simulink model "MPC"  (R2024b)
settings: Solver=ode4  StartTime=0.0  StopTime=tsim  FixedStep=baseRate  RelTol=1e-6  AbsTol=1e-6
values from neighbouring files (symbols this model uses):
  IBLACK = 0.1996    [unpackData.m]
  IRED = 0.1982    [unpackData.m]
  m = m + 5    (= 4)    [unpackData.m]
  M = diag([1/m; 1/m; 1/I])    [unpackData.m]
  mBLACK = 11.3620    (= 11.362)    [unpackData.m]
  mRED = 11.2970    (= 11.297)    [unpackData.m]
  N = 0    [unpackData.m]
  Q = blkdiag(0.0001*eye(2), 0.00001)    [unpackData.m]
  R = diag([6;6;6])    [unpackData.m]
undefined symbols (not defined in the file or in its folder): a1, a2, a3, alpha, alpha_m, alpha_t, alphas, alphas_t, alphat, Am, b, b0, b1, b2, b3, baseRate, Bm, C, c, c1, c1t, c2, c2t, camera_FOV, camera_offset, Cm, d, dataRate, DiscIntNeverNeededParam, Dm, docking_face, docking_offset, drop_states_ARM, drop_states_BLACK, drop_states_BLUE, drop_states_RED, epsilon, epsilont, eta, F_black_X_nominal, F_black_Y_nominal, F_blue_X_nominal, F_blue_Y_nominal, F_max, F_red_X_nominal, F_red_Y_nominal, f_t, F_t, F_thrusters_BLACK, F_thrusters_BLUE, F_thrusters_RED, F_u, f_u, F_v, gamma, Gamma1_el, Gamma1_sh, Gamma1_wr, Gamma2_el, Gamma2_sh ... (+118)
libraries: simulink x33, nvidiaSharedBlocks x13, slpidlib x6, MainLibrary x5, dspsigops x3, dspinverses x3, nvidiaIMUSensorslib x1
(part 5 of 11)

== system MPC/Thruster Control Code/Change BLUE Behavior ==
  note: Calculate the percentage of time each thruster must be on, and send to the PWM blocks.
  note: Using the attitude, rotate the forces into the body frame.
  note: Calculate which thrusters must be turned on and for how long.
  Action Port : ActionPort  ActionPortLabel=if(u1 == 3 | u2 == 1)
  Calculate Duty Cycle : Subsystem
  Data Store Read : DataStoreRead  DataStoreName=BLUE_Controls  IndexOptions=Index vector (dialog)  Indices=1  OutputSizes=1
  Data Store Read1 : DataStoreRead  DataStoreName=BLUE_Measured_States_RAW  IndexOptions=Index vector (dialog)  Indices=1  OutputSizes=1
  Data Store Write3 : DataStoreWrite  DataStoreName=BLUE_Saturated_Controls  IndexOptions=Index vector (dialog)  Indices=1  OutputSizes=1
  Demux : Demux  Outputs=[2,1]
  Demux1 : Demux  Outputs=[2,1,6]
  Mux1 : Mux  Inputs=2
  Rotate Forces to Body : Subsystem
  Terminator : Terminator
  Terminator1 : Terminator
  BLUE DC : Outport  VectorParamsAs1DForOutWhenUnconnected=off
  wires:
  Calculate Duty Cycle/1(Duty Cycle) -> BLUE DC/1
  Rotate Forces to Body/1(F_b) -> Mux1/1
  Demux/2 -> Mux1/2
  Mux1/1 -> Calculate Duty Cycle/1("[Fx_b; Fy_b; Tz]")
  Calculate Duty Cycle/2(Saturated Forces Moments) -> Data Store Write3/1
  Data Store Read/1 -> Demux/1
  Demux/1 -> Rotate Forces to Body/1("F_I ")
  Data Store Read1/1 -> Demux1/1
  Demux1/2 -> Calculate Duty Cycle/2(Measured Attitude), Rotate Forces to Body/2(Rz)
  Demux1/1 -> Terminator/1
  Demux1/3 -> Terminator1/1

== system MPC/Thruster Control Code/Change RED Behavior ==
  note: Calculate which thrusters must be turned on and for how long.
  note: Calculate the percentage of time each thruster must be on, and send to the PWM blocks.
  note: Using the attitude, rotate the forces into the body frame.
  Action Port : ActionPort  ActionPortLabel=if(u1 == 1 | u2 == 1)
  Calculate Duty Cycle : Subsystem
  Data Store Read : DataStoreRead  DataStoreName=RED_Controls  IndexOptions=Index vector (dialog)  Indices=1  OutputSizes=1
  Data Store Read2 : DataStoreRead  DataStoreName=RED_Measured_States_RAW  IndexOptions=Index vector (dialog)  Indices=1  OutputSizes=1
  Data Store Write1 : DataStoreWrite  DataStoreName=RED_Saturated_Controls  IndexOptions=Index vector (dialog)  Indices=1  OutputSizes=1
  Demux : Demux  Outputs=[2,1]
  Demux1 : Demux  Outputs=[2,1,6]
  Mux1 : Mux  Inputs=2
  Rotate Forces to Body : Subsystem
  Terminator : Terminator
  Terminator1 : Terminator
  RED DC : Outport  VectorParamsAs1DForOutWhenUnconnected=off
  wires:
  Demux/1 -> Rotate Forces to Body/1("F_I ")
  Mux1/1 -> Calculate Duty Cycle/1("[Fx_b; Fy_b; Tz]")
  Demux/2 -> Mux1/2
  Demux1/2 -> Calculate Duty Cycle/2(Measured Attitude), Rotate Forces to Body/2(Rz)
  Rotate Forces to Body/1(F_b) -> Mux1/1
  Data Store Read/1 -> Demux/1
  Demux1/1 -> Terminator/1
  Demux1/3 -> Terminator1/1
  Data Store Read2/1 -> Demux1/1
  Calculate Duty Cycle/2(Saturated Forces Moments) -> Data Store Write1/1
  Calculate Duty Cycle/1(Duty Cycle) -> RED DC/1

== system MPC/1 - Experiment Logic/Phase #2: Initial Position/Desired Joint Angles RED ==
  Constant1 : Constant  Value=pi/2
  Constant2 : Constant  Value=0
  Constant3 : Constant  Value=pi/2
  Mux : Mux  Inputs=3
  Target Array : Outport
  wires:
  Mux/1 -> Target Array/1
  Constant3/1 -> Mux/1
  Constant1/1 -> Mux/2
  Constant2/1 -> Mux/3

== system MPC/1 - Experiment Logic/Phase #2: Initial Position/Desired Position BLACK ==
  Desired States (BLACK) : Constant  Value=init_states_BLACK  SampleTime=-1
  Target Array : Outport
  wires:
  Desired States (BLACK)/1 -> Target Array/1

== system MPC/1 - Experiment Logic/Phase #2: Initial Position/Desired Position BLUE ==
  Desired States (BLUE) : Constant  Value=init_states_BLUE  SampleTime=-1
  Target Array : Outport
  wires:
  Desired States (BLUE)/1 -> Target Array/1

== system MPC/1 - Experiment Logic/Phase #2: Initial Position/Desired Position RED ==
  Constant2 : Constant  Value=init_states_RED
  Target Array : Outport
  wires:
  Constant2/1 -> Target Array/1

== system MPC/1 - Experiment Logic/Phase #3: Experiment/Sub-Phase #1 ==
  note: Experiment Logic (BLUE)
  note: Experiment Logic (Robotic Manipulator)
  note: Experiment Logic (RED)
  note: Experiment Logic (BLACK)
  note: Control Blocks
  Action Port : ActionPort  ActionPortLabel=if(u1 < u2)
  Constant : Constant  Value=[0 0 0]
  Constant1 : Constant  Value=[0 0 0]
  Constant{11..12,14..15,18} (5 alike) : Constant  Value=0
  Constant4 : Constant  Value=2
  Constant5 : Constant  Value=3
  Constant6 : Constant
  Constant8 : Constant  Value=2
  Data Store Write1 : DataStoreWrite  DataStoreName=ARM_Path_Planner_Selection  IndexOptions=Index vector (dialog)  Indices=1  OutputSizes=1
  Data Store Write10 : DataStoreWrite  DataStoreName=Toggle_Nav  IndexOptions=Index vector (dialog)  Indices=1  OutputSizes=1
  Data Store Write13 : DataStoreWrite  DataStoreName=ARM_Desired_States  IndexOptions=Index vector (dialog)  Indices=1  OutputSizes=1
  Data Store Write16 : DataStoreWrite  DataStoreName=BLUE_Control_Law_Enabler  IndexOptions=Index vector (dialog)  Indices=1  OutputSizes=1
  Data Store Write18 : DataStoreWrite  DataStoreName=BLUE_Desired_States  IndexOptions=Index vector (dialog)  Indices=1  OutputSizes=1
  Data Store Write2 : DataStoreWrite  DataStoreName=ARM_Control_Law_Enabler  IndexOptions=Index vector (dialog)  Indices=1  OutputSizes=1
  Data Store Write22 : DataStoreWrite  DataStoreName=BLUE_Path_Planner_Selection  IndexOptions=Index vector (dialog)  Indices=1  OutputSizes=1
  Data Store Write23 : DataStoreWrite  DataStoreName=BLACK_Path_Planner_Selection  IndexOptions=Index vector (dialog)  Indices=1  OutputSizes=1
  Data Store Write24 : DataStoreWrite  DataStoreName=RED_Path_Planner_Selection  IndexOptions=Index vector (dialog)  Indices=1  OutputSizes=1
  Data Store Write3 : DataStoreWrite  DataStoreName=RED_Control_Law_Enabler  IndexOptions=Index vector (dialog)  Indices=1  OutputSizes=1
  Data Store Write4 : DataStoreWrite  DataStoreName=BLACK_Control_Law_Enabler  IndexOptions=Index vector (dialog)  Indices=1  OutputSizes=1
  Data Store Write5 : DataStoreWrite  DataStoreName=BLACK_Desired_States  IndexOptions=Index vector (dialog)  Indices=1  OutputSizes=1
  Data Store Write7 : DataStoreWrite  DataStoreName=Float_State  IndexOptions=Index vector (dialog)  Indices=1  OutputSizes=1
  Data Store Write9 : DataStoreWrite  DataStoreName=RED_Desired_States  IndexOptions=Index vector (dialog)  Indices=1  OutputSizes=1
  Desired Position BLACK : Subsystem
  Desired Position BLUE : Subsystem
  Puck State1 : Constant
  wires:
  Desired Position BLACK/1(Target Array) -> Data Store Write5/1
  Desired Position BLUE/1(Target Array) -> Data Store Write18/1
  Constant/1 -> Data Store Write9/1
  Constant1/1 -> Data Store Write13/1
  Constant12/1 -> Data Store Write1/1
  Constant18/1 -> Data Store Write2/1
  Constant8/1 -> Data Store Write16/1
  Constant6/1 -> Data Store Write7/1
  Constant14/1 -> Data Store Write23/1
  Constant11/1 -> Data Store Write24/1
  Constant5/1 -> Data Store Write3/1
  Constant4/1 -> Data Store Write4/1
  Constant15/1 -> Data Store Write22/1
  Puck State1/1 -> Data Store Write10/1

== system MPC/1 - Experiment Logic/Phase #3: Experiment/Sub-Phase #2  ==
  note: Experiment Logic (BLACK)
  note: Experiment Logic (Robotic Manipulator)
  note: Experiment Logic (BLUE)
  note: Experiment Logic (RED)
  note: Control Blocks
  Action Port : ActionPort  ActionPortLabel=elseif((u1 < u3 & u1 >= u2))
  Constant : Constant  Value=[0 0 0]
  Constant1 : Constant  Value=[0 0 0]
  Constant{4,8,11..12,14..15,18} (7 alike) : Constant  Value=0
  Constant2 : Constant  Value=[0 0 0]
  Constant5 : Constant  Value=3
  Constant6 : Constant
  Data Store Write1 : DataStoreWrite  DataStoreName=ARM_Path_Planner_Selection  IndexOptions=Index vector (dialog)  Indices=1  OutputSizes=1
  Data Store Write10 : DataStoreWrite  DataStoreName=Toggle_Nav  IndexOptions=Index vector (dialog)  Indices=1  OutputSizes=1
  Data Store Write13 : DataStoreWrite  DataStoreName=ARM_Desired_States  IndexOptions=Index vector (dialog)  Indices=1  OutputSizes=1
  Data Store Write16 : DataStoreWrite  DataStoreName=BLUE_Control_Law_Enabler  IndexOptions=Index vector (dialog)  Indices=1  OutputSizes=1
  Data Store Write18 : DataStoreWrite  DataStoreName=BLUE_Desired_States  IndexOptions=Index vector (dialog)  Indices=1  OutputSizes=1
  Data Store Write2 : DataStoreWrite  DataStoreName=ARM_Control_Law_Enabler  IndexOptions=Index vector (dialog)  Indices=1  OutputSizes=1
  Data Store Write22 : DataStoreWrite  DataStoreName=BLUE_Path_Planner_Selection  IndexOptions=Index vector (dialog)  Indices=1  OutputSizes=1
  Data Store Write23 : DataStoreWrite  DataStoreName=BLACK_Path_Planner_Selection  IndexOptions=Index vector (dialog)  Indices=1  OutputSizes=1
  Data Store Write24 : DataStoreWrite  DataStoreName=RED_Path_Planner_Selection  IndexOptions=Index vector (dialog)  Indices=1  OutputSizes=1
  Data Store Write3 : DataStoreWrite  DataStoreName=RED_Control_Law_Enabler  IndexOptions=Index vector (dialog)  Indices=1  OutputSizes=1
  Data Store Write4 : DataStoreWrite  DataStoreName=BLACK_Control_Law_Enabler  IndexOptions=Index vector (dialog)  Indices=1  OutputSizes=1
  Data Store Write5 : DataStoreWrite  DataStoreName=BLACK_Desired_States  IndexOptions=Index vector (dialog)  Indices=1  OutputSizes=1
  Data Store Write7 : DataStoreWrite  DataStoreName=Float_State  IndexOptions=Index vector (dialog)  Indices=1  OutputSizes=1
  Data Store Write9 : DataStoreWrite  DataStoreName=RED_Desired_States  IndexOptions=Index vector (dialog)  Indices=1  OutputSizes=1
  Desired Position BLACK : Subsystem
  Puck State1 : Constant
  wires:
  Constant/1 -> Data Store Write9/1
  Desired Position BLACK/1(Target Array) -> Data Store Write5/1
  Constant2/1 -> Data Store Write18/1
  Constant1/1 -> Data Store Write13/1
  Constant15/1 -> Data Store Write22/1
  Constant4/1 -> Data Store Write4/1
  Constant8/1 -> Data Store Write16/1
  Constant18/1 -> Data Store Write2/1
  Constant6/1 -> Data Store Write7/1
  Constant11/1 -> Data Store Write24/1
  Constant5/1 -> Data Store Write3/1
  Constant12/1 -> Data Store Write1/1
  Constant14/1 -> Data Store Write23/1
  Puck State1/1 -> Data Store Write10/1

== system MPC/1 - Experiment Logic/Phase #3: Experiment/Sub-Phase #3  ==
  note: Experiment Logic (BLACK)
  note: Experiment Logic (Robotic Manipulator)
  note: Experiment Logic (BLUE)
  note: Experiment Logic (RED)
  note: Control Blocks
  Action Port : ActionPort  ActionPortLabel=elseif((u1 < u4 & u1 >= u3))
  Constant : Constant  Value=[0 0 0]
  Constant1 : Constant  Value=[0 0 0]
  Constant{4,8,11..12,14..15,18} (7 alike) : Constant  Value=0
  Constant2 : Constant  Value=[0 0 0]
  Constant5 : Constant  Value=3
  Constant6 : Constant
  Data Store Write1 : DataStoreWrite  DataStoreName=ARM_Path_Planner_Selection  IndexOptions=Index vector (dialog)  Indices=1  OutputSizes=1
  Data Store Write10 : DataStoreWrite  DataStoreName=Toggle_Nav  IndexOptions=Index vector (dialog)  Indices=1  OutputSizes=1
  Data Store Write13 : DataStoreWrite  DataStoreName=ARM_Desired_States  IndexOptions=Index vector (dialog)  Indices=1  OutputSizes=1
  Data Store Write16 : DataStoreWrite  DataStoreName=BLUE_Control_Law_Enabler  IndexOptions=Index vector (dialog)  Indices=1  OutputSizes=1
  Data Store Write18 : DataStoreWrite  DataStoreName=BLUE_Desired_States  IndexOptions=Index vector (dialog)  Indices=1  OutputSizes=1
  Data Store Write2 : DataStoreWrite  DataStoreName=ARM_Control_Law_Enabler  IndexOptions=Index vector (dialog)  Indices=1  OutputSizes=1
  Data Store Write22 : DataStoreWrite  DataStoreName=BLUE_Path_Planner_Selection  IndexOptions=Index vector (dialog)  Indices=1  OutputSizes=1
  Data Store Write23 : DataStoreWrite  DataStoreName=BLACK_Path_Planner_Selection  IndexOptions=Index vector (dialog)  Indices=1  OutputSizes=1
  Data Store Write24 : DataStoreWrite  DataStoreName=RED_Path_Planner_Selection  IndexOptions=Index vector (dialog)  Indices=1  OutputSizes=1
  Data Store Write3 : DataStoreWrite  DataStoreName=RED_Control_Law_Enabler  IndexOptions=Index vector (dialog)  Indices=1  OutputSizes=1
  Data Store Write4 : DataStoreWrite  DataStoreName=BLACK_Control_Law_Enabler  IndexOptions=Index vector (dialog)  Indices=1  OutputSizes=1
  Data Store Write5 : DataStoreWrite  DataStoreName=BLACK_Desired_States  IndexOptions=Index vector (dialog)  Indices=1  OutputSizes=1
  Data Store Write7 : DataStoreWrite  DataStoreName=Float_State  IndexOptions=Index vector (dialog)  Indices=1  OutputSizes=1
  Data Store Write9 : DataStoreWrite  DataStoreName=RED_Desired_States  IndexOptions=Index vector (dialog)  Indices=1  OutputSizes=1
  Desired Position BLACK : Subsystem
  Puck State1 : Constant
  wires:
  Constant/1 -> Data Store Write9/1
  Desired Position BLACK/1(Target Array) -> Data Store Write5/1
  Constant2/1 -> Data Store Write18/1
  Constant1/1 -> Data Store Write13/1
  Constant12/1 -> Data Store Write1/1
  Constant14/1 -> Data Store Write23/1
  Constant4/1 -> Data Store Write4/1
  Constant8/1 -> Data Store Write16/1
  Constant15/1 -> Data Store Write22/1
  Constant6/1 -> Data Store Write7/1
  Constant18/1 -> Data Store Write2/1
  Constant11/1 -> Data Store Write24/1
  Constant5/1 -> Data Store Write3/1
  Puck State1/1 -> Data Store Write10/1

== system MPC/1 - Experiment Logic/Phase #3: Experiment/Sub-Phase #4 ==
  note: Experiment Logic (BLACK)
  note: Experiment Logic (Robotic Manipulator)
  note: Experiment Logic (BLUE)
  note: Experiment Logic (RED)
  note: Control Blocks
  Action Port : ActionPort  ActionPortLabel=elseif( (u1 < u5 & u1 >= u4))
  Constant : Constant  Value=[0 0 0]
  Constant1 : Constant  Value=[0 0 0]
  Constant{8,11..12,14..15,18} (6 alike) : Constant  Value=0
  Constant2 : Constant  Value=[0 0 0]
  Constant4 : Constant
  Constant5 : Constant
  Constant6 : Constant
  Data Store Write1 : DataStoreWrite  DataStoreName=ARM_Path_Planner_Selection  IndexOptions=Index vector (dialog)  Indices=1  OutputSizes=1
  Data Store Write10 : DataStoreWrite  DataStoreName=Toggle_Nav  IndexOptions=Index vector (dialog)  Indices=1  OutputSizes=1
  Data Store Write13 : DataStoreWrite  DataStoreName=ARM_Desired_States  IndexOptions=Index vector (dialog)  Indices=1  OutputSizes=1
  Data Store Write16 : DataStoreWrite  DataStoreName=BLUE_Control_Law_Enabler  IndexOptions=Index vector (dialog)  Indices=1  OutputSizes=1
  Data Store Write18 : DataStoreWrite  DataStoreName=BLUE_Desired_States  IndexOptions=Index vector (dialog)  Indices=1  OutputSizes=1
  Data Store Write2 : DataStoreWrite  DataStoreName=ARM_Control_Law_Enabler  IndexOptions=Index vector (dialog)  Indices=1  OutputSizes=1
  Data Store Write22 : DataStoreWrite  DataStoreName=BLUE_Path_Planner_Selection  IndexOptions=Index vector (dialog)  Indices=1  OutputSizes=1
  Data Store Write23 : DataStoreWrite  DataStoreName=BLACK_Path_Planner_Selection  IndexOptions=Index vector (dialog)  Indices=1  OutputSizes=1
  Data Store Write24 : DataStoreWrite  DataStoreName=RED_Path_Planner_Selection  IndexOptions=Index vector (dialog)  Indices=1  OutputSizes=1
  Data Store Write3 : DataStoreWrite  DataStoreName=RED_Control_Law_Enabler  IndexOptions=Index vector (dialog)  Indices=1  OutputSizes=1
  Data Store Write4 : DataStoreWrite  DataStoreName=BLACK_Control_Law_Enabler  IndexOptions=Index vector (dialog)  Indices=1  OutputSizes=1
  Data Store Write5 : DataStoreWrite  DataStoreName=BLACK_Desired_States  IndexOptions=Index vector (dialog)  Indices=1  OutputSizes=1
  Data Store Write7 : DataStoreWrite  DataStoreName=Float_State  IndexOptions=Index vector (dialog)  Indices=1  OutputSizes=1
  Data Store Write9 : DataStoreWrite  DataStoreName=RED_Desired_States  IndexOptions=Index vector (dialog)  Indices=1  OutputSizes=1
  Desired Position BLACK : Subsystem
  Puck State1 : Constant  Value=0
  wires:
  Constant/1 -> Data Store Write9/1
  Desired Position BLACK/1(Target Array) -> Data Store Write5/1
  Constant2/1 -> Data Store Write18/1
  Constant1/1 -> Data Store Write13/1
  Constant14/1 -> Data Store Write23/1
  Constant18/1 -> Data Store Write2/1
  Constant11/1 -> Data Store Write24/1
  Constant4/1 -> Data Store Write4/1
  Constant15/1 -> Data Store Write22/1
  Constant8/1 -> Data Store Write16/1
  Constant5/1 -> Data Store Write3/1
  Constant6/1 -> Data Store Write7/1
  Constant12/1 -> Data Store Write1/1
  Puck State1/1 -> Data Store Write10/1

== system MPC/1 - Experiment Logic/Phase #4: Return Home/Desired Joint Angles RED ==
  Constant1 : Constant  Value=pi/2
  Constant2 : Constant  Value=0
  Constant3 : Constant  Value=pi/2
  Mux : Mux  Inputs=3
  Target Array : Outport
  wires:
  Mux/1 -> Target Array/1
  Constant3/1 -> Mux/1
  Constant1/1 -> Mux/2
  Constant2/1 -> Mux/3

== system MPC/1 - Experiment Logic/Phase #4: Return Home/Desired Position BLACK ==
  Desired States (BLACK) : Constant  Value=home_states_BLACK  SampleTime=-1
  Target Array : Outport
  wires:
  Desired States (BLACK)/1 -> Target Array/1

== system MPC/1 - Experiment Logic/Phase #4: Return Home/Desired Position BLUE ==
  Desired States (BLUE) : Constant  Value=home_states_BLUE  SampleTime=-1
  Target Array : Outport
  wires:
  Desired States (BLUE)/1 -> Target Array/1

== system MPC/1 - Experiment Logic/Phase #4: Return Home/Desired Position RED ==
  Constant2 : Constant  Value=home_states_RED
  Target Array : Outport
  wires:
  Constant2/1 -> Target Array/1

== system MPC/1 - Experiment Logic/Phase #5: Hold Home/Desired Joint Angles RED ==
  Constant1 : Constant  Value=pi/2
  Constant2 : Constant  Value=0
  Constant3 : Constant  Value=pi/2
  Mux : Mux  Inputs=3
  Target Array : Outport
  wires:
  Mux/1 -> Target Array/1
  Constant3/1 -> Mux/1
  Constant1/1 -> Mux/2
  Constant2/1 -> Mux/3

== system MPC/1 - Experiment Logic/Phase #5: Hold Home/Desired Position BLACK ==
  Desired States (BLACK) : Constant  Value=home_states_BLACK  SampleTime=-1
  Target Array : Outport
  wires:
  Desired States (BLACK)/1 -> Target Array/1

== system MPC/1 - Experiment Logic/Phase #5: Hold Home/Desired Position BLUE ==
  Desired States (BLUE) : Constant  Value=home_states_BLUE  SampleTime=-1
  Target Array : Outport
  wires:
  Desired States (BLUE)/1 -> Target Array/1

== system MPC/1 - Experiment Logic/Phase #5: Hold Home/Desired Position RED ==
  Constant2 : Constant  Value=home_states_RED
  Target Array : Outport
  wires:
  Constant2/1 -> Target Array/1

== system MPC/2 - Guidance/Custom PPL (ARM)/Desired Position ==
  Data Store Read : DataStoreRead  DataStoreName=ARM_Desired_States  IndexOptions=Index vector (dialog)  Indices=1  OutputSizes=1
  Position Array : Outport
  wires:
  Data Store Read/1 -> Position Array/1

== system MPC/2 - Guidance/Custom PPL (BLACK)/Desired Position ==
  BLACK_Px : DataStoreRead  DataStoreName=BLACK_Desired_States  IndexOptions=Index vector (dialog)  Indices=1  OutputSizes=1
  Position Array : Outport
  wires:
  BLACK_Px/1 -> Position Array/1

== system MPC/2 - Guidance/Custom PPL (BLUE)/Desired Position ==
  Data Store Read4 : DataStoreRead  DataStoreName=BLUE_Desired_States  IndexOptions=Index vector (dialog)  Indices=1  OutputSizes=1
  Position Array : Outport
  wires:
  Data Store Read4/1 -> Position Array/1

== system MPC/2 - Guidance/Custom PPL (RED)/Desired Position ==
  RED_Px : DataStoreRead  DataStoreName=RED_Desired_States  IndexOptions=Index vector (dialog)  Indices=1  OutputSizes=1
  Position Array : Outport
  wires:
  RED_Px/1 -> Position Array/1

== system MPC/2 - Guidance/Default APF PPL (BLACK)/Current Position RED ==
  Demux : Demux  Outputs=[3,6]
  RED_Px : DataStoreRead  DataStoreName=BLACK_Measured_States  IndexOptions=Index vector (dialog)  Indices=1  OutputSizes=1
  Terminator : Terminator
  Position Array : Outport
  wires:
  RED_Px/1 -> Demux/1
  Demux/1 -> Position Array/1
  Demux/2 -> Terminator/1

== system MPC/2 - Guidance/Default APF PPL (BLACK)/Obstacles ==
  Current Position BLUE : Subsystem
  Current Position RED : Subsystem
  Matrix Concatenate : Concatenate  Mode=Multidimensional array
  Obstacle Positions : Outport
  wires:
  Current Position RED/1(Position Array) -> Matrix Concatenate/2
  Current Position BLUE/1(Position Array) -> Matrix Concatenate/1
  Matrix Concatenate/1 -> Obstacle Positions/1

== system MPC/2 - Guidance/Default APF PPL (RED)/Current Position RED ==
  Data Store Read2 : DataStoreRead  DataStoreName=RED_Measured_States  IndexOptions=Index vector (dialog)  Indices=1  OutputSizes=1
  Demux : Demux  Outputs=[3,6]
  Terminator : Terminator
  Position Array : Outport
  wires:
  Data Store Read2/1 -> Demux/1
  Demux/1 -> Position Array/1
  Demux/2 -> Terminator/1

== system MPC/2 - Guidance/Default APF PPL (RED)/Obstacles ==
  Current Position BLACK : Subsystem
  Current Position BLUE : Subsystem
  Matrix Concatenate : Concatenate  Mode=Multidimensional array
  Obstacle Positions : Outport
  wires:
  Current Position BLACK/1(Position Array) -> Matrix Concatenate/2
  Current Position BLUE/1(Position Array) -> Matrix Concatenate/1
  Matrix Concatenate/1 -> Obstacle Positions/1

== system MPC/2 - Guidance/Disable PPL (ARM)/Desired Position ==
  Data Store Read : DataStoreRead  DataStoreName=ARM_Desired_States  IndexOptions=Index vector (dialog)  Indices=1  OutputSizes=1
  Position Array : Outport
  wires:
  Data Store Read/1 -> Position Array/1

== system MPC/2 - Guidance/Disable PPL (BLACK)/Desired Position ==
  BLACK_Px : DataStoreRead  DataStoreName=BLACK_Desired_States  IndexOptions=Index vector (dialog)  Indices=1  OutputSizes=1
  Position Array : Outport
  wires:
  BLACK_Px/1 -> Position Array/1

== system MPC/2 - Guidance/Disable PPL (BLUE)/Desired Position ==
  Data Store Read4 : DataStoreRead  DataStoreName=BLUE_Desired_States  IndexOptions=Index vector (dialog)  Indices=1  OutputSizes=1
  Position Array : Outport
  wires:
  Data Store Read4/1 -> Position Array/1

== system MPC/2 - Guidance/Disable PPL (RED)/Desired Position ==
  RED_Px : DataStoreRead  DataStoreName=RED_Desired_States  IndexOptions=Index vector (dialog)  Indices=1  OutputSizes=1
  Position Array : Outport
  wires:
  RED_Px/1 -> Position Array/1

== system MPC/3 - Navigation/Subsystem/DQMEKF ==
  Data Store Read : DataStoreRead  DataStoreName=dt  IndexOptions=Index vector (dialog)  Indices=1  OutputSizes=1
  Data Store Read1 : DataStoreRead  DataStoreName=Vis_dq  IndexOptions=Index vector (dialog)  Indices=1  OutputSizes=1
  Data Store Read2 : DataStoreRead  DataStoreName=Red_dq  IndexOptions=Index vector (dialog)  Indices=1  OutputSizes=1
  Data Store Write1 : DataStoreWrite  DataStoreName=DQMEKFerror  IndexOptions=Index vector (dialog)  Indices=1  OutputSizes=1
  Data Store Write17 : DataStoreWrite  DataStoreName=DQMEKFx  IndexOptions=Index vector (dialog)  Indices=1  OutputSizes=1
  Data Store Write18 : DataStoreWrite  DataStoreName=DQMEKFP  IndexOptions=Index vector (dialog)  Indices=1  OutputSizes=1
  Data Store Write19 : DataStoreWrite  DataStoreName=DQMEKFt  IndexOptions=Index vector (dialog)  Indices=1  OutputSizes=1
  Data Store Write2 : DataStoreWrite  DataStoreName=DQMEKFNIS  IndexOptions=Index vector (dialog)  Indices=1  OutputSizes=1
  Delay : Delay  DelayLength=1  InitialCondition=PDQ
  Delay1 : Delay  DelayLength=1  InitialCondition=[1;zeros(13,1)]
  MATLAB Function1 : MATLAB Function  TreatAsAtomicUnit=on
  MATLAB Function3 : MATLAB Function  TreatAsAtomicUnit=on
  wires:
  Delay/1 -> MATLAB Function1/5(P_prev)
  Delay1/1 -> MATLAB Function1/4(x_prev)
  Data Store Read/1 -> MATLAB Function1/1(dt)
  Data Store Read1/1 -> MATLAB Function1/3(VIS_dq)
  Data Store Read2/1 -> MATLAB Function1/2(RED_dq)
  MATLAB Function1/5(NIS) -> Data Store Write2/1  "NIS"
  MATLAB Function1/2(P_est) -> Delay/1, Data Store Write18/1
  MATLAB Function1/3(compT) -> Data Store Write19/1
  MATLAB Function1/1(x_est) -> Delay1/1, MATLAB Function3/1(u)
  MATLAB Function3/1(x) -> Data Store Write17/1
  MATLAB Function1/4(y) -> Data Store Write1/1

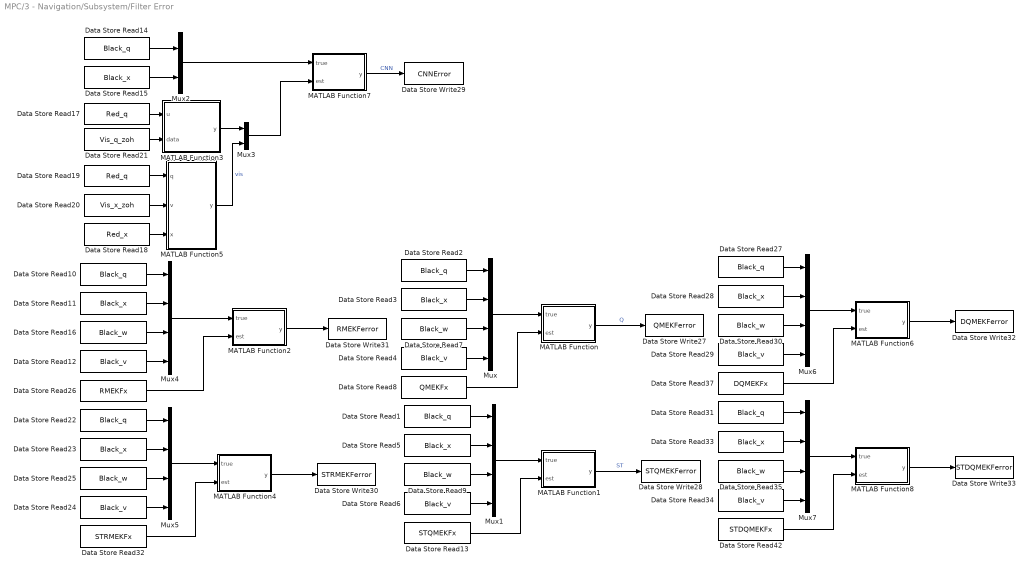
== system MPC/3 - Navigation/Subsystem/Filter Error ==
  Data Store Read{1..2,10,14,22,27,31} (7 alike) : DataStoreRead  DataStoreName=Black_q  IndexOptions=Index vector (dialog)  Indices=1  OutputSizes=1
  Data Store Read{3,5,11,15,23,28,33} (7 alike) : DataStoreRead  DataStoreName=Black_x  IndexOptions=Index vector (dialog)  Indices=1  OutputSizes=1
  Data Store Read{4,6,12,24,29,34} (6 alike) : DataStoreRead  DataStoreName=Black_v  IndexOptions=Index vector (dialog)  Indices=1  OutputSizes=1
  Data Store Read13 : DataStoreRead  DataStoreName=STQMEKFx  IndexOptions=Index vector (dialog)  Indices=1  OutputSizes=1
  Data Store Read{7,9,16,25,30,35} (6 alike) : DataStoreRead  DataStoreName=Black_w  IndexOptions=Index vector (dialog)  Indices=1  OutputSizes=1
  Data Store Read17 : DataStoreRead  DataStoreName=Red_q  IndexOptions=Index vector (dialog)  Indices=1  OutputSizes=1
  Data Store Read18 : DataStoreRead  DataStoreName=Red_x  IndexOptions=Index vector (dialog)  Indices=1  OutputSizes=1
  Data Store Read19 : DataStoreRead  DataStoreName=Red_q  IndexOptions=Index vector (dialog)  Indices=1  OutputSizes=1
  Data Store Read20 : DataStoreRead  DataStoreName=Vis_x_zoh  IndexOptions=Index vector (dialog)  Indices=1  OutputSizes=1
  Data Store Read21 : DataStoreRead  DataStoreName=Vis_q_zoh  IndexOptions=Index vector (dialog)  Indices=1  OutputSizes=1
  Data Store Read26 : DataStoreRead  DataStoreName=RMEKFx  IndexOptions=Index vector (dialog)  Indices=1  OutputSizes=1
  Data Store Read32 : DataStoreRead  DataStoreName=STRMEKFx  IndexOptions=Index vector (dialog)  Indices=1  OutputSizes=1
  Data Store Read37 : DataStoreRead  DataStoreName=DQMEKFx  IndexOptions=Index vector (dialog)  Indices=1  OutputSizes=1
  Data Store Read42 : DataStoreRead  DataStoreName=STDQMEKFx  IndexOptions=Index vector (dialog)  Indices=1  OutputSizes=1
  Data Store Read8 : DataStoreRead  DataStoreName=QMEKFx  IndexOptions=Index vector (dialog)  Indices=1  OutputSizes=1
  Data Store Write27 : DataStoreWrite  DataStoreName=QMEKFerror  IndexOptions=Index vector (dialog)  Indices=1  OutputSizes=1
  Data Store Write28 : DataStoreWrite  DataStoreName=STQMEKFerror  IndexOptions=Index vector (dialog)  Indices=1  OutputSizes=1
  Data Store Write29 : DataStoreWrite  DataStoreName=CNNError  IndexOptions=Index vector (dialog)  Indices=1  OutputSizes=1
  Data Store Write30 : DataStoreWrite  DataStoreName=STRMEKFerror  IndexOptions=Index vector (dialog)  Indices=1  OutputSizes=1
  Data Store Write31 : DataStoreWrite  DataStoreName=RMEKFerror  IndexOptions=Index vector (dialog)  Indices=1  OutputSizes=1
  Data Store Write32 : DataStoreWrite  DataStoreName=DQMEKFerror  IndexOptions=Index vector (dialog)  Indices=1  OutputSizes=1
  Data Store Write33 : DataStoreWrite  DataStoreName=STDQMEKFerror  IndexOptions=Index vector (dialog)  Indices=1  OutputSizes=1
  MATLAB Function : MATLAB Function  TreatAsAtomicUnit=on
  MATLAB Function1 : MATLAB Function  TreatAsAtomicUnit=on
  MATLAB Function2 : MATLAB Function  TreatAsAtomicUnit=on
  MATLAB Function3 : MATLAB Function  TreatAsAtomicUnit=on
  MATLAB Function4 : MATLAB Function  TreatAsAtomicUnit=on
  MATLAB Function5 : MATLAB Function  TreatAsAtomicUnit=on
  MATLAB Function6 : MATLAB Function  TreatAsAtomicUnit=on
  MATLAB Function7 : MATLAB Function  TreatAsAtomicUnit=on
  MATLAB Function8 : MATLAB Function  TreatAsAtomicUnit=on
  Mux{,1,4..7} (6 alike) : Mux
  Mux2 : Mux  Inputs=2
  Mux3 : Mux  Inputs=2
  wires:
  Data Store Read20/1 -> MATLAB Function5/2(v)
  MATLAB Function8/1(y) -> Data Store Write33/1
  Data Store Read17/1 -> MATLAB Function3/1(u)
  Data Store Read14/1 -> Mux2/1
  Mux3/1 -> MATLAB Function7/2(est)
  Data Store Read8/1 -> MATLAB Function/2(est)
  MATLAB Function2/1(y) -> Data Store Write31/1
  MATLAB Function/1(y) -> Data Store Write27/1  "Q"
  Data Store Read32/1 -> MATLAB Function4/2(est)
  Data Store Read2/1 -> Mux/1
  MATLAB Function7/1(y) -> Data Store Write29/1  "CNN"
  Mux2/1 -> MATLAB Function7/1(true)
  Mux1/1 -> MATLAB Function1/1(true)
  MATLAB Function6/1(y) -> Data Store Write32/1
  Mux5/1 -> MATLAB Function4/1(true)
  MATLAB Function3/1(y) -> Mux3/1
  Mux/1 -> MATLAB Function/1(true)
  Mux4/1 -> MATLAB Function2/1(true)
  Data Store Read4/1 -> Mux/4
  Mux6/1 -> MATLAB Function6/1(true)
  Data Store Read18/1 -> MATLAB Function5/3(x)
  Mux7/1 -> MATLAB Function8/1(true)
  MATLAB Function4/1(y) -> Data Store Write30/1
  MATLAB Function5/1(y) -> Mux3/2  "vis"
  Data Store Read19/1 -> MATLAB Function5/1(q)
  Data Store Read42/1 -> MATLAB Function8/2(est)
  Data Store Read13/1 -> MATLAB Function1/2(est)
  Data Store Read21/1 -> MATLAB Function3/2(data)
  Data Store Read26/1 -> MATLAB Function2/2(est)
  MATLAB Function1/1(y) -> Data Store Write28/1  "ST"
  Data Store Read15/1 -> Mux2/2
  Data Store Read37/1 -> MATLAB Function6/2(est)
  Data Store Read7/1 -> Mux/3
  Data Store Read3/1 -> Mux/2
  Data Store Read5/1 -> Mux1/2
  Data Store Read1/1 -> Mux1/1
  Data Store Read6/1 -> Mux1/4
  Data Store Read9/1 -> Mux1/3
  Data Store Read11/1 -> Mux4/2
  Data Store Read10/1 -> Mux4/1
  Data Store Read12/1 -> Mux4/4
  Data Store Read16/1 -> Mux4/3
  Data Store Read23/1 -> Mux5/2
  Data Store Read22/1 -> Mux5/1
  Data Store Read24/1 -> Mux5/4
  Data Store Read25/1 -> Mux5/3
  Data Store Read28/1 -> Mux6/2
  Data Store Read27/1 -> Mux6/1
  Data Store Read29/1 -> Mux6/4
  Data Store Read30/1 -> Mux6/3
  Data Store Read33/1 -> Mux7/2
  Data Store Read31/1 -> Mux7/1
  Data Store Read34/1 -> Mux7/4
  Data Store Read35/1 -> Mux7/3

== system MPC/3 - Navigation/Subsystem/QMEKF ==
  Data Store Read : DataStoreRead  DataStoreName=dt  IndexOptions=Index vector (dialog)  Indices=1  OutputSizes=1
  Data Store Read1 : DataStoreRead  DataStoreName=Red_q  IndexOptions=Index vector (dialog)  Indices=1  OutputSizes=1
  Data Store Read2 : DataStoreRead  DataStoreName=Red_x  IndexOptions=Index vector (dialog)  Indices=1  OutputSizes=1
  Data Store Read3 : DataStoreRead  DataStoreName=Vis_q  IndexOptions=Index vector (dialog)  Indices=1  OutputSizes=1
  Data Store Read4 : DataStoreRead  DataStoreName=Vis_x  IndexOptions=Index vector (dialog)  Indices=1  OutputSizes=1
  Data Store Write1 : DataStoreWrite  DataStoreName=QMEKFerror  IndexOptions=Index vector (dialog)  Indices=1  OutputSizes=1
  Data Store Write17 : DataStoreWrite  DataStoreName=QMEKFx  IndexOptions=Index vector (dialog)  Indices=1  OutputSizes=1
  Data Store Write18 : DataStoreWrite  DataStoreName=QMEKFP  IndexOptions=Index vector (dialog)  Indices=1  OutputSizes=1
  Data Store Write19 : DataStoreWrite  DataStoreName=QMEKFt  IndexOptions=Index vector (dialog)  Indices=1  OutputSizes=1
  Data Store Write2 : DataStoreWrite  DataStoreName=QMEKFNIS  IndexOptions=Index vector (dialog)  Indices=1  OutputSizes=1
  Delay : Delay  DelayLength=1  InitialCondition=PQ
  Delay1 : Delay  DelayLength=1  InitialCondition=[1;zeros(12,1)]
  MATLAB Function : MATLAB Function  TreatAsAtomicUnit=on
  MATLAB Function1 : MATLAB Function  TreatAsAtomicUnit=on
  wires:
  Delay/1 -> MATLAB Function1/7(P_prev)
  MATLAB Function1/2(P_est) -> Delay/1, Data Store Write18/1
  Delay1/1 -> MATLAB Function1/6(x_prev)
  MATLAB Function1/1(x_est) -> MATLAB Function/1(u), Delay1/1
  MATLAB Function1/3(compT) -> Data Store Write19/1
  Data Store Read/1 -> MATLAB Function1/1(dt)
  Data Store Read1/1 -> MATLAB Function1/2(RED_quat)
  Data Store Read2/1 -> MATLAB Function1/3(RED_x)
  Data Store Read3/1 -> MATLAB Function1/4(BLACK_q)
  Data Store Read4/1 -> MATLAB Function1/5(BLACK_x)
  MATLAB Function/1(out) -> Data Store Write17/1
  MATLAB Function1/5(NIS) -> Data Store Write2/1  "NIS"
  MATLAB Function1/4(y) -> Data Store Write1/1

== system MPC/3 - Navigation/Subsystem/RMEKF ==
  Data Store Read : DataStoreRead  DataStoreName=dt  IndexOptions=Index vector (dialog)  Indices=1  OutputSizes=1
  Data Store Read15 : DataStoreRead  DataStoreName=Vis_R  IndexOptions=Index vector (dialog)  Indices=1  OutputSizes=1
  Data Store Read2 : DataStoreRead  DataStoreName=Red_x  IndexOptions=Index vector (dialog)  Indices=1  OutputSizes=1
  Data Store Read3 : DataStoreRead  DataStoreName=Red_q  IndexOptions=Index vector (dialog)  Indices=1  OutputSizes=1
  Data Store Read4 : DataStoreRead  DataStoreName=Vis_x  IndexOptions=Index vector (dialog)  Indices=1  OutputSizes=1
  Data Store Write1 : DataStoreWrite  DataStoreName=RMEKFR  IndexOptions=Index vector (dialog)  Indices=1  OutputSizes=1
  Data Store Write17 : DataStoreWrite  DataStoreName=RMEKFx  IndexOptions=Index vector (dialog)  Indices=1  OutputSizes=1
  Data Store Write18 : DataStoreWrite  DataStoreName=RMEKFP  IndexOptions=Index vector (dialog)  Indices=1  OutputSizes=1
  Data Store Write19 : DataStoreWrite  DataStoreName=RMEKFt  IndexOptions=Index vector (dialog)  Indices=1  OutputSizes=1
  Data Store Write2 : DataStoreWrite  DataStoreName=RMEKFerror  IndexOptions=Index vector (dialog)  Indices=1  OutputSizes=1
  Data Store Write6 : DataStoreWrite  DataStoreName=RMEKFNIS  IndexOptions=Index vector (dialog)  Indices=1  OutputSizes=1
  Delay : Delay  DelayLength=1  InitialCondition=PR
  Delay1 : Delay  DelayLength=1  InitialCondition=zeros(9,1)
  Delay2 : Delay  DelayLength=1  InitialCondition=eye(3)
  MATLAB Function : MATLAB Function  TreatAsAtomicUnit=on
  MATLAB Function1 : MATLAB Function  TreatAsAtomicUnit=on
  MATLAB Function11 : MATLAB Function  TreatAsAtomicUnit=on
  wires:
  Delay/1 -> MATLAB Function1/8(P_prev)
  MATLAB Function1/3(P_est) -> Delay/1, Data Store Write18/1
  Delay1/1 -> MATLAB Function1/6(x_prev)
  MATLAB Function1/1(x_est) -> Delay1/1, MATLAB Function/1(x)
  MATLAB Function1/4(compT) -> Data Store Write19/1
  Data Store Read/1 -> MATLAB Function1/1(dt)
  Data Store Read3/1 -> MATLAB Function1/2(RED_yaw)
  Data Store Read2/1 -> MATLAB Function1/3(RED_x)
  Data Store Read15/1 -> MATLAB Function1/4(VIS_R)
  Data Store Read4/1 -> MATLAB Function1/5(VIS_x)
  MATLAB Function1/2(Rot_est) -> Delay2/1, Data Store Write1/1, MATLAB Function11/1(u)
  Delay2/1 -> MATLAB Function1/7(Rot_prev)
  MATLAB Function11/1(y) -> MATLAB Function/2(q)  "q"
  MATLAB Function/1(out) -> Data Store Write17/1
  MATLAB Function1/6(NIS) -> Data Store Write6/1  "NIS"
  MATLAB Function1/5(y) -> Data Store Write2/1

== system MPC/3 - Navigation/Subsystem/Representations ==
  u : Inport
  MATLAB Function : MATLAB Function  TreatAsAtomicUnit=on
  dq : Outport
  q : Outport  Port=2
  R : Outport  Port=3
  x : Outport  Port=4
  v : Outport  Port=5
  w : Outport  Port=6
  yaw : Outport  Port=7
  wires:
  u/1 -> MATLAB Function/1(u)
  MATLAB Function/1(dq) -> dq/1
  MATLAB Function/2(q) -> q/1
  MATLAB Function/3(R) -> R/1
  MATLAB Function/4(x) -> x/1
  MATLAB Function/5(v) -> v/1
  MATLAB Function/6(w) -> w/1
  MATLAB Function/7(yaw) -> yaw/1

== system MPC/3 - Navigation/Subsystem/Representations1 ==
  u : Inport
  MATLAB Function : MATLAB Function  TreatAsAtomicUnit=on
  dq : Outport
  q : Outport  Port=2
  R : Outport  Port=3
  x : Outport  Port=4
  v : Outport  Port=5
  w : Outport  Port=6
  yaw : Outport  Port=7
  wires:
  u/1 -> MATLAB Function/1(u)
  MATLAB Function/1(dq) -> dq/1
  MATLAB Function/2(q) -> q/1
  MATLAB Function/3(R) -> R/1
  MATLAB Function/4(x) -> x/1
  MATLAB Function/5(v) -> v/1
  MATLAB Function/6(w) -> w/1
  MATLAB Function/7(yaw) -> yaw/1

== system MPC/3 - Navigation/Subsystem/STDQMEKF ==
  Data Store Read : DataStoreRead  DataStoreName=dt  IndexOptions=Index vector (dialog)  Indices=1  OutputSizes=1
  Data Store Read1 : DataStoreRead  DataStoreName=Vis_dq  IndexOptions=Index vector (dialog)  Indices=1  OutputSizes=1
  Data Store Read2 : DataStoreRead  DataStoreName=Red_dq  IndexOptions=Index vector (dialog)  Indices=1  OutputSizes=1
  Data Store Write1 : DataStoreWrite  DataStoreName=STDQMEKFerror  IndexOptions=Index vector (dialog)  Indices=1  OutputSizes=1
  Data Store Write17 : DataStoreWrite  DataStoreName=STDQMEKFx  IndexOptions=Index vector (dialog)  Indices=1  OutputSizes=1
  Data Store Write18 : DataStoreWrite  DataStoreName=STDQMEKFP  IndexOptions=Index vector (dialog)  Indices=1  OutputSizes=1
  Data Store Write19 : DataStoreWrite  DataStoreName=STDQMEKFt  IndexOptions=Index vector (dialog)  Indices=1  OutputSizes=1
  Data Store Write2 : DataStoreWrite  DataStoreName=STDQMEKFNIS  IndexOptions=Index vector (dialog)  Indices=1  OutputSizes=1
  Delay : Delay  DelayLength=1  InitialCondition=PDQ
  Delay1 : Delay  DelayLength=1  InitialCondition=[1;zeros(13,1)]
  Delay2 : Delay  DelayLength=1  InitialCondition=zeros(6)
  MATLAB Function1 : MATLAB Function  TreatAsAtomicUnit=on
  MATLAB Function3 : MATLAB Function  TreatAsAtomicUnit=on
  wires:
  Delay/1 -> MATLAB Function1/5(P_prev)
  Delay1/1 -> MATLAB Function1/4(x_prev)
  MATLAB Function1/1(x_est) -> Delay1/1, MATLAB Function3/1(u)
  Data Store Read/1 -> MATLAB Function1/1(dt)
  MATLAB Function1/6(V_est) -> Delay2/1
  Delay2/1 -> MATLAB Function1/6(V_prev)
  Data Store Read2/1 -> MATLAB Function1/2(RED_dq)
  Data Store Read1/1 -> MATLAB Function1/3(VIS_dq)
  MATLAB Function1/3(compT) -> Data Store Write19/1
  MATLAB Function3/1(x) -> Data Store Write17/1
  MATLAB Function1/2(P_est) -> Delay/1, Data Store Write18/1
  MATLAB Function1/4(y) -> Data Store Write1/1
  MATLAB Function1/5(NIS) -> Data Store Write2/1

== system MPC/3 - Navigation/Subsystem/STQMEKF ==
  Data Store Read : DataStoreRead  DataStoreName=dt  IndexOptions=Index vector (dialog)  Indices=1  OutputSizes=1
  Data Store Read1 : DataStoreRead  DataStoreName=Red_q  IndexOptions=Index vector (dialog)  Indices=1  OutputSizes=1
  Data Store Read2 : DataStoreRead  DataStoreName=Red_x  IndexOptions=Index vector (dialog)  Indices=1  OutputSizes=1
  Data Store Read3 : DataStoreRead  DataStoreName=Vis_q  IndexOptions=Index vector (dialog)  Indices=1  OutputSizes=1
  Data Store Read4 : DataStoreRead  DataStoreName=Vis_x  IndexOptions=Index vector (dialog)  Indices=1  OutputSizes=1
  Data Store Write1 : DataStoreWrite  DataStoreName=STQMEKFerror  IndexOptions=Index vector (dialog)  Indices=1  OutputSizes=1
  Data Store Write17 : DataStoreWrite  DataStoreName=STQMEKFx  IndexOptions=Index vector (dialog)  Indices=1  OutputSizes=1
  Data Store Write18 : DataStoreWrite  DataStoreName=STQMEKFP  IndexOptions=Index vector (dialog)  Indices=1  OutputSizes=1
  Data Store Write19 : DataStoreWrite  DataStoreName=STQMEKFt  IndexOptions=Index vector (dialog)  Indices=1  OutputSizes=1
  Data Store Write2 : DataStoreWrite  DataStoreName=STQMEKFNIS  IndexOptions=Index vector (dialog)  Indices=1  OutputSizes=1
  Delay : Delay  DelayLength=1  InitialCondition=PQ
  Delay1 : Delay  DelayLength=1  InitialCondition=[1;zeros(12,1)]
  Delay2 : Delay  DelayLength=1  InitialCondition=zeros(6)
  MATLAB Function1 : MATLAB Function  TreatAsAtomicUnit=on
  MATLAB Function2 : MATLAB Function  TreatAsAtomicUnit=on
  wires:
  Delay/1 -> MATLAB Function1/7(P_prev)
  MATLAB Function1/2(P_est) -> Delay/1, Data Store Write18/1
  Delay1/1 -> MATLAB Function1/6(x_prev)
  MATLAB Function1/1(x_est) -> MATLAB Function2/1(u), Delay1/1
  Data Store Read/1 -> MATLAB Function1/1(dt)
  Data Store Read1/1 -> MATLAB Function1/2(RED_quat)
  Data Store Read2/1 -> MATLAB Function1/3(RED_x)
  Data Store Read3/1 -> MATLAB Function1/4(BLACK_q)
  Data Store Read4/1 -> MATLAB Function1/5(BLACK_x)
  MATLAB Function1/6(V_est) -> Delay2/1
  Delay2/1 -> MATLAB Function1/8(V_prev)
  MATLAB Function2/1(out) -> Data Store Write17/1
  MATLAB Function1/4(y) -> Data Store Write1/1
  MATLAB Function1/5(NIS) -> Data Store Write2/1  "NIS"
  MATLAB Function1/3(compT) -> Data Store Write19/1

== system MPC/3 - Navigation/Subsystem/STRMEKF ==
  Data Store Read : DataStoreRead  DataStoreName=dt  IndexOptions=Index vector (dialog)  Indices=1  OutputSizes=1
  Data Store Read1 : DataStoreRead  DataStoreName=Vis_R  IndexOptions=Index vector (dialog)  Indices=1  OutputSizes=1
  Data Store Read2 : DataStoreRead  DataStoreName=Red_x  IndexOptions=Index vector (dialog)  Indices=1  OutputSizes=1
  Data Store Read3 : DataStoreRead  DataStoreName=Red_q  IndexOptions=Index vector (dialog)  Indices=1  OutputSizes=1
  Data Store Read4 : DataStoreRead  DataStoreName=Vis_x  IndexOptions=Index vector (dialog)  Indices=1  OutputSizes=1
  Data Store Write1 : DataStoreWrite  DataStoreName=STRMEKFR  IndexOptions=Index vector (dialog)  Indices=1  OutputSizes=1
  Data Store Write17 : DataStoreWrite  DataStoreName=STRMEKFx  IndexOptions=Index vector (dialog)  Indices=1  OutputSizes=1
  Data Store Write18 : DataStoreWrite  DataStoreName=STRMEKFP  IndexOptions=Index vector (dialog)  Indices=1  OutputSizes=1
  Data Store Write19 : DataStoreWrite  DataStoreName=STRMEKFt  IndexOptions=Index vector (dialog)  Indices=1  OutputSizes=1
  Data Store Write2 : DataStoreWrite  DataStoreName=STRMEKFerror  IndexOptions=Index vector (dialog)  Indices=1  OutputSizes=1
  Data Store Write6 : DataStoreWrite  DataStoreName=STRMEKFNIS  IndexOptions=Index vector (dialog)  Indices=1  OutputSizes=1
  Delay1 : Delay  DelayLength=1  InitialCondition=zeros(9,1)
  Delay2 : Delay  DelayLength=1  InitialCondition=PR
  Delay3 : Delay  DelayLength=1  InitialCondition=zeros(6)
  Delay4 : Delay  DelayLength=1  InitialCondition=eye(3)
  MATLAB Function : MATLAB Function  TreatAsAtomicUnit=on
  MATLAB Function1 : MATLAB Function  TreatAsAtomicUnit=on
  MATLAB Function11 : MATLAB Function  TreatAsAtomicUnit=on
  wires:
  Data Store Read/1 -> MATLAB Function1/1(dt)
  Data Store Read3/1 -> MATLAB Function1/2(RED_yaw)
  Data Store Read2/1 -> MATLAB Function1/3(RED_x)
  Data Store Read1/1 -> MATLAB Function1/4(VIS_R)
  Data Store Read4/1 -> MATLAB Function1/5(VIS_x)
  Delay2/1 -> MATLAB Function1/8(P_prev)
  Delay1/1 -> MATLAB Function1/6(x_prev)
  Delay3/1 -> MATLAB Function1/9(V_prev)
  MATLAB Function1/7(V_est) -> Delay3/1
  Delay4/1 -> MATLAB Function1/7(Rot_prev)
  MATLAB Function1/6(NIS) -> Data Store Write6/1  "NIS"
  MATLAB Function1/5(y) -> Data Store Write2/1
  MATLAB Function/1(out) -> Data Store Write17/1
  MATLAB Function1/3(P_est) -> Delay2/1, Data Store Write18/1
  MATLAB Function1/1(x_est) -> Delay1/1, MATLAB Function/1(x)
  MATLAB Function1/4(compT) -> Data Store Write19/1
  MATLAB Function1/2(Rot_est) -> Delay4/1, MATLAB Function11/1(u), Data Store Write1/1
  MATLAB Function11/1(y) -> MATLAB Function/2(q)  "q"

== system MPC/4 - Control/Default LQR Control (BLACK)/Calculate Error ==
  Desired Attitude : Inport
  Measured Attitude : Inport  Port=2
  MATLAB Function : MATLAB Function  TreatAsAtomicUnit=on
  Attitude Error : Outport
  wires:
  MATLAB Function/1(Rz_error) -> Attitude Error/1
  Desired Attitude/1 -> MATLAB Function/1(Rz_path)
  Measured Attitude/1 -> MATLAB Function/2(Rz_measured)

== system MPC/4 - Control/Default LQR Control (BLUE)/Calculate Error ==
  Desired Attitude : Inport
  Measured Attitude : Inport  Port=2
  MATLAB Function : MATLAB Function  TreatAsAtomicUnit=on
  Attitude Error : Outport
  wires:
  MATLAB Function/1(Rz_error) -> Attitude Error/1
  Desired Attitude/1 -> MATLAB Function/1(Rz_path)
  Measured Attitude/1 -> MATLAB Function/2(Rz_measured)

== system MPC/4 - Control/Default LQR Control (RED)/Calculate Error ==
  Desired Attitude : Inport
  Measured Attitude : Inport  Port=2
  MATLAB Function : MATLAB Function  TreatAsAtomicUnit=on
  Attitude Error : Outport
  wires:
  MATLAB Function/1(Rz_error) -> Attitude Error/1
  Desired Attitude/1 -> MATLAB Function/1(Rz_path)
  Measured Attitude/1 -> MATLAB Function/2(Rz_measured)

== system MPC/4 - Control/Default PD (ARM)/Passthrough for Experiment ==
  q1_desired : Inport
  q2_desired : Inport  Port=2
  q3_desired : Inport  Port=3
  Action Port : ActionPort  ActionPortLabel=else
  q1_command : Outport
  q2_command : Outport  Port=2
  q3_command : Outport  Port=3
  wires:
  q3_desired/1 -> q3_command/1
  q1_desired/1 -> q1_command/1
  q2_desired/1 -> q2_command/1

== system MPC/4 - Control/Default PD (ARM)/Simulated Position Controller ==
  q1_desired : Inport
  q2_desired : Inport  Port=2
  q3_desired : Inport  Port=3
  Action Port : ActionPort  ActionPortLabel=if(u1 == 1)
  Custom Discrete PD (Elbow) : Subsystem
  Custom Discrete PD (Shoulder) : Subsystem
  Custom Discrete PD (Wrist) : Subsystem
  Data Store Read2 : DataStoreRead  DataStoreName=ARM_Measured_States  IndexOptions=Index vector (dialog)  Indices=1  OutputSizes=1
  Demux : Demux  Outputs=[1,1,1,3]
  Saturation : Saturate  UpperLimit=Tz_lim_sharm  LowerLimit=-Tz_lim_sharm
  Saturation1 : Saturate  UpperLimit=Tz_lim_elarm  LowerLimit=-Tz_lim_elarm
  Saturation3 : Saturate  UpperLimit=Tz_lim_wrarm  LowerLimit=-Tz_lim_wrarm
  Subtract2 : Sum  Inputs=+-
  Subtract3 : Sum  Inputs=+-
  Subtract4 : Sum  Inputs=+-
  Terminator : Terminator
  q1_command : Outport
  q2_command : Outport  Port=2
  q3_command : Outport  Port=3
  wires:
  Saturation3/1 -> q3_command/1
  Subtract4/1 -> Custom Discrete PD (Wrist)/1(ey)
  Custom Discrete PD (Shoulder)/1(Fx) -> Saturation/1
  Custom Discrete PD (Elbow)/1(Fy) -> Saturation1/1
  Saturation/1 -> q1_command/1
  Subtract2/1 -> Custom Discrete PD (Shoulder)/1(ex)
  Saturation1/1 -> q2_command/1
  Custom Discrete PD (Wrist)/1(Fy) -> Saturation3/1
  Subtract3/1 -> Custom Discrete PD (Elbow)/1(ey)
  Demux/1 -> Subtract2/2
  Demux/2 -> Subtract3/2
  Demux/3 -> Subtract4/2
  q1_desired/1 -> Subtract2/1
  q2_desired/1 -> Subtract3/1
  q3_desired/1 -> Subtract4/1
  Data Store Read2/1 -> Demux/1
  Demux/4 -> Terminator/1

== system MPC/4 - Control/Default PD Control (BLACK)/Calculate Error ==
  Desired Attitude : Inport
  Measured Attitude : Inport  Port=2
  MATLAB Function : MATLAB Function  TreatAsAtomicUnit=on
  Attitude Error : Outport
  wires:
  MATLAB Function/1(Rz_error) -> Attitude Error/1
  Desired Attitude/1 -> MATLAB Function/1(Rz_path)
  Measured Attitude/1 -> MATLAB Function/2(Rz_measured)

== system MPC/4 - Control/Default PD Control (BLUE)/Calculate Error ==
  Desired Attitude : Inport
  Measured Attitude : Inport  Port=2
  MATLAB Function : MATLAB Function  TreatAsAtomicUnit=on
  Attitude Error : Outport
  wires:
  MATLAB Function/1(Rz_error) -> Attitude Error/1
  Desired Attitude/1 -> MATLAB Function/1(Rz_path)
  Measured Attitude/1 -> MATLAB Function/2(Rz_measured)

== system MPC/4 - Control/Default PD Control (RED)/CSMC ==
  In1 : Inport
  Demux : Demux  Outputs=3
  MATLAB Function : MATLAB Function  TreatAsAtomicUnit=on
  MATLAB Function1 : MATLAB Function  TreatAsAtomicUnit=on
  MATLAB Function2 : MATLAB Function  TreatAsAtomicUnit=on
  MATLAB Function3 : MATLAB Function  TreatAsAtomicUnit=on
  MATLAB Function4 : MATLAB Function  TreatAsAtomicUnit=on
  MATLAB Function5 : MATLAB Function  TreatAsAtomicUnit=on
  MATLAB Function6 : MATLAB Function  TreatAsAtomicUnit=on
  MATLAB Function7 : MATLAB Function  TreatAsAtomicUnit=on
  MATLAB Function8 : MATLAB Function  TreatAsAtomicUnit=on
  Mux : Mux  Inputs=3
  Pseudo Derivative : DiscreteTransferFcn  Numerator=[N, -N]  Denominator=[1, -1 + N*Ts]
  Pseudo Derivative1 : DiscreteTransferFcn  Numerator=[N, -N]  Denominator=[1, -1 + N*Ts]
  Pseudo Derivative2 : DiscreteTransferFcn  Numerator=[N, -N]  Denominator=[1, -1 + N*Ts]
  Saturation{,1..4} (5 alike) : Saturate  UpperLimit=epsilon  LowerLimit=-epsilon
  Saturation5 : Saturate  UpperLimit=epsilont  LowerLimit=-epsilont
  Sum : Sum  Inputs=++|
  Sum1 : Sum  Inputs=++|
  Sum2 : Sum  Inputs=++|
  Out1 : Outport
  wires:
  Demux/1 -> MATLAB Function2/1(q1), Pseudo Derivative/1
  Pseudo Derivative/1 -> MATLAB Function2/2(q2), MATLAB Function1/1(q2)
  Sum/1 -> Mux/1
  MATLAB Function/1(u) -> Saturation1/1
  MATLAB Function1/1(u) -> Saturation/1
  MATLAB Function2/1(phi) -> MATLAB Function/1(phi)
  Saturation/1 -> Sum/2
  Saturation1/1 -> Sum/1
  Saturation2/1 -> Sum1/2
  MATLAB Function5/1(phi) -> MATLAB Function3/1(phi)
  Saturation3/1 -> Sum1/1
  Demux/2 -> MATLAB Function5/1(q1), Pseudo Derivative1/1
  Pseudo Derivative1/1 -> MATLAB Function4/1(q2), MATLAB Function5/2(q2)
  MATLAB Function4/1(u) -> Saturation2/1
  MATLAB Function3/1(u) -> Saturation3/1
  Sum1/1 -> Mux/2
  Demux/3 -> Pseudo Derivative2/1, MATLAB Function8/1(q1)
  MATLAB Function7/1(u) -> Saturation4/1
  Saturation4/1 -> Sum2/2
  Saturation5/1 -> Sum2/1
  Pseudo Derivative2/1 -> MATLAB Function7/1(q2), MATLAB Function8/2(q2)
  MATLAB Function8/1(phi) -> MATLAB Function6/1(phi)
  MATLAB Function6/1(u) -> Saturation5/1
  Sum2/1 -> Mux/3
  Mux/1 -> Out1/1
  In1/1 -> Demux/1
